simulink library "mbed_targets_stm_disco_f407"  (R2015a)
settings: Solver=ode45  StartTime=0.0  StopTime=10.0  RelTol=1e-3
libraries: mbed_lib x8
settings Model: CovSFcnEnable=off  Creator=oh  LastModifiedBy=oh
settings DebuggingCC: SolverPrmCheckMsg=warning

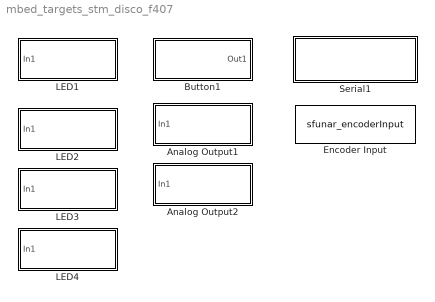
== system mbed_targets_stm_disco_f407 ==
  Analog Output1 : Subsystem  mask{Parameter1=0}
      mask Display:
      | offset=0.7;
      | plot([0+offset:0.025:0.25+offset],0.3*sin(2*pi*[0:0.1:1])+0.5)
      | port_label('input',1,['DAC1 (PA.4)']);
  Analog Output2 : Subsystem
      mask Display:
      | offset=0.7;
      | plot([0+offset:0.025:0.25+offset],0.3*sin(2*pi*[0:0.1:1])+0.5)
      | port_label('input',1,['DAC2 (PA.5)']);
  Button1 : Subsystem  mask{Parameter1=0}
      mask Display:
      | plot([0 0.15 0.15 0.35 0.35 0.5],[0.3 0.3 0.7 0.7 0.3 0.3])
      | port_label('output',1,['UsrBtn1']);
  Encoder Input : S-Function  FunctionName=sfunar_encoderInput  Parameters=SampleTime, uint8(TimerNumber), uint8(EncoderMode), uint8(Ti1Port), uint8(Ti1Pin), uint8(Ti2Port), uint8(Ti2Pin), uint8(InputMode), uint16(Resolution)  mask{TimerNumber=TIM1, EncoderMode=TI1, Ti1Port=A, Ti1Pin=0, Ti2Port=A, Ti2Pin=0, InputMode=PullNone, Resolution=65535, SampleTime=-1}
      mask prompts: TimerNumber "Timer number:"; EncoderMode "Encoder Mode:"; Ti1Port "TI1 Port"; Ti1Pin "TI1 Pin"; Ti2Port "TI2 Port"; Ti2Pin "TI2 Pin"; InputMode "Input Mode (GPIO):"; Resolution "Resolution (Pulses/Rev):"; SampleTime "Sample time: (-1 for inherited)"
      mask TypeOptions TimerNumber: TIM1 | TIM2 | TIM3 | TIM4 | TIM5 | TIM8
      mask TypeOptions EncoderMode: TI1 | TI2 | TI1 and TI2
      mask TypeOptions Ti1Port: A | B | C | D | E | F
      mask TypeOptions Ti1Pin: 0 | 1 | 2 | 3 | 4 | 5 | 6 | 7 | 8 | 9 | 10 | 11 | 12 | 13 | 14 | 15
      mask TypeOptions Ti2Port: A | B | C | D | E | F
      mask TypeOptions Ti2Pin: 0 | 1 | 2 | 3 | 4 | 5 | 6 | 7 | 8 | 9 | 10 | 11 | 12 | 13 | 14 | 15
      mask TypeOptions InputMode: PullNone | PullUp | PullDown
      mask DialogControl DescTextVar Prompt: Hardware Encoder für STM32F4xx
      mask Display:
      | port_label('input',1,'Reset');
      | disp(['Timer ' num2str(TimerNumber) '\n\n']);
      | disp(['\nTI1:P' Ti1Port+64 '.' num2str(Ti1Pin-1) '\n' 'TI2:P' Ti2Port+64 '.' num2str(Ti2Pin-1) ]);
      | port_label('output',1,'Angle');
      | port_label('output',2,'RAW');
  LED1 : Subsystem  mask{Parameter1=0}
      mask Display:
      | plot([0.5 0.65 0.65 0.85 0.85 1],[0.3 0.3 0.7 0.7 0.3 0.3])
      | port_label('input',1,['LED1']);
  LED2 : Subsystem  mask{Parameter1=0}
      mask Display:
      | plot([0.5 0.65 0.65 0.85 0.85 1],[0.3 0.3 0.7 0.7 0.3 0.3])
      | port_label('input',1,['LED2']);
  LED3 : Subsystem  mask{Parameter1=0}
      mask Display:
      | plot([0.5 0.65 0.65 0.85 0.85 1],[0.3 0.3 0.7 0.7 0.3 0.3])
      | port_label('input',1,['LED3']);
  LED4 : Subsystem  mask{Parameter1=0}
      mask Display:
      | plot([0.5 0.65 0.65 0.85 0.85 1],[0.3 0.3 0.7 0.7 0.3 0.3])
      | port_label('input',1,['LED4']);
  Serial1 : Subsystem  mask{Parameter1=0}
      mask Display: disp(['Serial1(USB)\nTX:PA_2, RX:PA_3'])

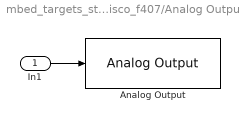
== system mbed_targets_stm_disco_f407/Analog Output1 ==
  In1 : Inport
  Analog Output : mbed_lib/GPIO/Analog Output  SParameter2=A  SParameter1=4  inputVariant=Double: 0 - 1.0f  SampleTime=-1
  wires:
  In1/1 -> Analog Output/1

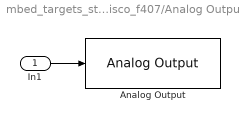
== system mbed_targets_stm_disco_f407/Analog Output2 ==
  In1 : Inport
  Analog Output : mbed_lib/GPIO/Analog Output  SParameter2=A  SParameter1=5  inputVariant=Double: 0 - 1.0f  SampleTime=-1
  wires:
  In1/1 -> Analog Output/1

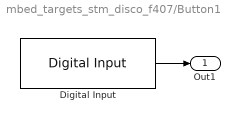
== system mbed_targets_stm_disco_f407/Button1 ==
  Digital Input : mbed_lib/GPIO/Digital Input  SParameter2=A  SParameter1=0  SParameter3=PullDefault  SampleTime=-1
  Out1 : Outport
  wires:
  Digital Input/1 -> Out1/1

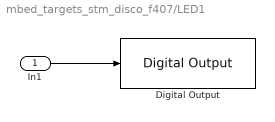
== system mbed_targets_stm_disco_f407/LED1 ==
  In1 : Inport
  Digital Output : mbed_lib/GPIO/Digital Output  SParameter2=D  SParameter1=12  SParameter3=PullDefault  SampleTime=-1
  wires:
  In1/1 -> Digital Output/1

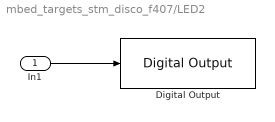
== system mbed_targets_stm_disco_f407/LED2 ==
  In1 : Inport
  Digital Output : mbed_lib/GPIO/Digital Output  SParameter2=D  SParameter1=13  SParameter3=PullDefault  SampleTime=-1
  wires:
  In1/1 -> Digital Output/1

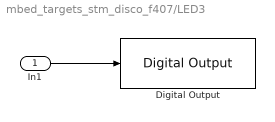
== system mbed_targets_stm_disco_f407/LED3 ==
  In1 : Inport
  Digital Output : mbed_lib/GPIO/Digital Output  SParameter2=D  SParameter1=14  SParameter3=PullDefault  SampleTime=-1
  wires:
  In1/1 -> Digital Output/1

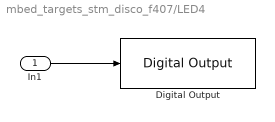
== system mbed_targets_stm_disco_f407/LED4 ==
  In1 : Inport
  Digital Output : mbed_lib/GPIO/Digital Output  SParameter2=D  SParameter1=15  SParameter3=PullDefault  SampleTime=-1
  wires:
  In1/1 -> Digital Output/1

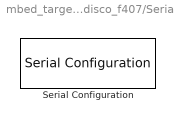
== system mbed_targets_stm_disco_f407/Serial1 ==
  Serial Configuration : mbed_lib/Serial/Serial Configuration  SerialPort=1  TXPort=A  TXPin=2  RXPort=A  RXPin=3  BaudRate=9600
